simulink model "example_QProblem"  (Simulink 7.4)
settings: Solver=FixedStepDiscrete  StartTime=0.0  StopTime=0.5  RelTol=1e-3
undefined symbols (not defined in the file or in its folder): A, H
settings Model: Creator=jferreau  LastModifiedBy=chjofer2  ExtModeAutoUpdateStatusClock=off
settings OptimizationCC: InitFltsAndDblsToZero=on
settings DebuggingCC: SaveWithParameterizedLinksMsg=none  SignalResolutionControl=TryResolveAllWithWarning
settings GRTTargetCC: TargetFcnLib=ansi_tfl_tmw.mat

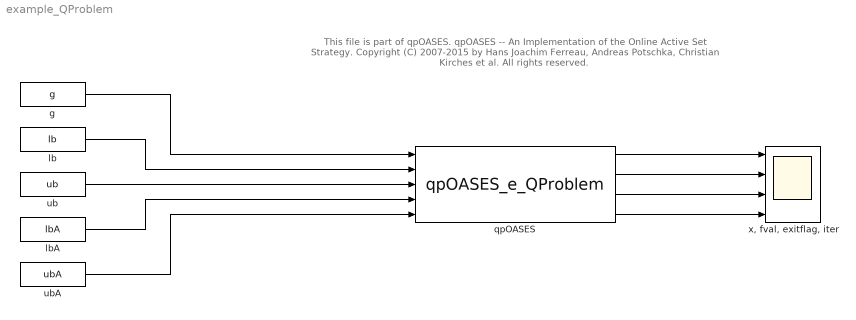
== system example_QProblem ==
  note: This file is part of qpOASES.
      |
      | qpOASES -- An Implementation of the Online Active Set Strategy.
      | Copyright (C) 2007-2015 by Hans Joachim Ferreau, Andreas Potschka, Christian Kirches et al.
      | All rights reserved.
  g : FromWorkspace  VariableName=g  SampleTime=0.1  OutputAfterFinalValue=Holding final value
  lb : FromWorkspace  VariableName=lb  SampleTime=0.1  OutputAfterFinalValue=Holding final value
  lbA : FromWorkspace  VariableName=lbA  SampleTime=0.1  OutputAfterFinalValue=Holding final value
  qpOASES : S-Function  FunctionName=qpOASES_e_QProblem  Parameters=H,A  EnableBusSupport=off
  ub : FromWorkspace  VariableName=ub  SampleTime=0.1  OutputAfterFinalValue=Holding final value
  ubA : FromWorkspace  VariableName=ubA  SampleTime=0.1  OutputAfterFinalValue=Holding final value
  "x, fval, exitflag, iter" : Scope  NumInputPorts=4
      settings: YMin=-5~-5~-5~-5  YMax=5~5~5~5
  wires:
  qpOASES/1 -> "x, fval, exitflag, iter"/1
  qpOASES/2 -> "x, fval, exitflag, iter"/2
  qpOASES/3 -> "x, fval, exitflag, iter"/3
  qpOASES/4 -> "x, fval, exitflag, iter"/4
  ub/1 -> qpOASES/3
  lb/1 -> qpOASES/2
  g/1 -> qpOASES/1
  lbA/1 -> qpOASES/4
  ubA/1 -> qpOASES/5
